simulink model "LRMate200Experimentor_Trq2DSA"  (R2015b)
settings: Solver=FixedStepDiscrete  StartTime=0.0  StopTime=10.0  FixedStep=si.SolverTimeStep  RelTol=1e-3
model workspace (MATLAB code in the model file):
  | rsi = evalin('base', 'si.ri{1}');
undefined symbols (not defined in the file or in its folder): si
settings Model: xpc_rtwmakecfg_data=_xpcethercatlib_  ParameterArgumentNames=rsi  Creator=rluser  LastModifiedBy=Chin
settings SolverCC: EnableConcurrentExecution=on
settings DataIOCC: SaveFormat=Array
settings OptimizationCC: BlockReduction=off  OptimizeBlockIOStorage=off  BufferReuse=off  GlobalBufferReuse=off  ExpressionFolding=off  LocalBlockOutputs=off
settings DebuggingCC: SolverPrmCheckMsg=warning
settings HardwareCC: ProdBitPerPointer=32  ProdLargestAtomicFloat=None  ProdWordSize=32  ProdLongLongMode=on  ProdHWDeviceType=Generic->32-bit x86 compatible
settings RTWCC: SystemTargetFile=slrt.tlc  TemplateMakefile=slrt_default_tmf  Description=Simulink Real-Time  RTWCompilerOptimization=on
settings CodeAppCC: MaxIdLength=120
settings SimulinkRealTimeCC: GeneratePreprocessorConditionals=Disable all
settings ConfigComp: CovModelRefEnable=Off  CovSFcnEnable=off

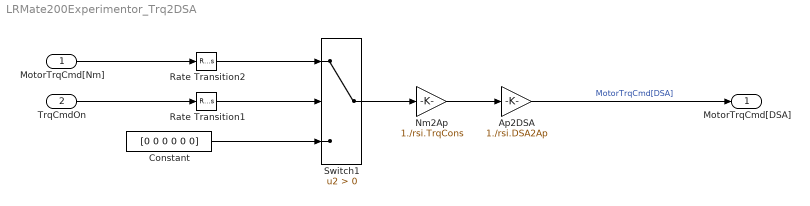
== system LRMate200Experimentor_Trq2DSA ==
  MotorTrqCmd[Nm] : Inport  PortDimensions=6
  TrqCmdOn : Inport  Port=2  OutDataTypeStr=boolean
  Ap2DSA : Gain  Gain=1./rsi.DSA2Ap
  Constant : Constant  Value=[0 0 0 0 0 0]  SampleTime=si.tsv
  Nm2Ap : Gain  Gain=1./rsi.TrqCons
  Rate Transition1 : RateTransition  OutPortSampleTime=si.tsv
  Rate Transition2 : RateTransition  OutPortSampleTime=si.tsv
  Switch1 : Switch  Criteria=u2 > Threshold
  MotorTrqCmd[DSA] : Outport
  wires:
  Constant/1 -> Switch1/3
  TrqCmdOn/1 -> Rate Transition1/1
  Rate Transition1/1 -> Switch1/2
  Switch1/1 -> Nm2Ap/1
  Nm2Ap/1 -> Ap2DSA/1
  Ap2DSA/1 -> MotorTrqCmd[DSA]/1  "MotorTrqCmd[DSA]"
  MotorTrqCmd[Nm]/1 -> Rate Transition2/1
  Rate Transition2/1 -> Switch1/1
